simulink model "VehDyn14DOF"  (R2024b)
settings: Solver=VariableStepAuto  StartTime=0.0  StopTime=inf  FixedStep=0.001  RelTol=1e-3
model workspace (MAT data in the model file):
  ssEnable : Simulink.Parameter (value not decoded)
  xdot_r : Simulink.Parameter (value not decoded)
values from neighbouring files (symbols this model uses):
  AccPwrbp = 0.0 3.0779560993538198    [vehDyn14DOF.sldd]
  AccSpdbp = 256.49641719585139 641.24104298962845    [vehDyn14DOF.sldd]
  Downshift_Speeds = 9.5625 12.9375 16.3125 19.6875 23.0625 26.4375 29.8125 33.1875 36.5625 39.9375 43.3125 46.687499999999986 47.8125 51.187499999999986 54.562499999999986 57.9375 59.0625 62.4375 65.8125 69.1875 68.90625 72.84375 76.78125 80.71875 78.75 83.25 87.75 92.25    [vehDyn14DOF.sldd]
  EngRevLim = 7000.0    [vehDyn14DOF.sldd]
  F0z = 2886.0 2907.0    [vehDyn14DOF.sldd]
  Pedal_Positions = 0.1 0.4 0.5 0.9    [vehDyn14DOF.sldd]
  Trans = 0.01    [vehDyn14DOF.sldd]
  Upshift_Speeds = 12.9375 16.3125 19.6875 33.0 26.4375 29.8125 33.1875 52.5 39.9375 43.3125 46.687499999999986 77.25 51.187499999999986 54.562499999999986 57.9375 100.5 62.4375 65.8125 69.1875 138.75 72.84375 76.78125 80.71875 161.875 83.25 87.75 92.25 185.0    [vehDyn14DOF.sldd]
  VEH = 1575.0    [vehDyn14DOF.sldd]
symbols that are objects in the model workspace (value not decoded): ssEnable, xdot_r
undefined symbols (not defined in the file or in its folder): AccelCmd, CurvGradRef, CurvRef, DecelCmd, DiscIntNeverNeededParam, egoVehDyn, EnblAccelCmd, EnblDecelCmd, EnblSteerCmd, GearCmd, Gnd, Iz, lambda_mux, lambda_muy, lf, LngRef, lr, LtrRef, m, max_dc, maxSteer, PhiRef, SteerCmd, steeringGain, SteerZero, Wind, XRef, YRef, Z
libraries: simulink x14, autolibutils x13, autolibsharedcoupling x11, vehdynlibtire x10, vehdynlibsuspension x8, sharedtransform x5, autolibshareddiff x5, shared6dof x2, slpidlib x1, autolibtranscontrolscommon x1, vehdynlibdriver x1, autolibshared x1
(part 3 of 10)

== system VehDyn14DOF/Passenger Vehicle/Engine Input ==
  Cntrl : Inport
  Driveline : Inport  Port=2
  Bus Selector : BusSelector  OutputSignals=ECU.EngTrqCmd
  Bus Selector1 : BusSelector  OutputSignals=EngSpd
  EngTrqCmd : Outport  VectorParamsAs1DForOutWhenUnconnected=off
  EngSpd : Outport  Port=2  VectorParamsAs1DForOutWhenUnconnected=off
  wires:
  Driveline/1 -> Bus Selector1/1
  Cntrl/1 -> Bus Selector/1
  Bus Selector/1 -> EngTrqCmd/1  "<EngTrqCmd>"
  Bus Selector1/1 -> EngSpd/1  "<EngSpd>"

== system VehDyn14DOF/Passenger Vehicle/Engine Output ==
  "EngTrq " : Inport
  Bus Creator : BusCreator  Inputs=1
  Eng : Outport  VectorParamsAs1DForOutWhenUnconnected=off
  wires:
  "EngTrq "/1 -> Bus Creator/1  "EngTrq"
  Bus Creator/1 -> Eng/1

== system VehDyn14DOF/Passenger Vehicle/Pedal Cluster Input ==
  Driver : Inport
  Driveline : Inport  Port=2
  Steering : Inport  Port=3
  Bus Selector : BusSelector  OutputSignals=steer_cmd,accel_cmd,decel_cmd,gear_cmd
  Bus Selector1 : BusSelector  OutputSignals=BrkPrs
  Bus Selector2 : BusSelector  OutputSignals=StrWhlTrq
  SteerCmd : Outport  VectorParamsAs1DForOutWhenUnconnected=off
  AccelCmd : Outport  Port=2  VectorParamsAs1DForOutWhenUnconnected=off
  DecelCmd : Outport  Port=3  VectorParamsAs1DForOutWhenUnconnected=off
  GearCmd : Outport  Port=4  VectorParamsAs1DForOutWhenUnconnected=off
  BrkPrs : Outport  Port=5  VectorParamsAs1DForOutWhenUnconnected=off
  StrWhlTrq : Outport  Port=6  VectorParamsAs1DForOutWhenUnconnected=off
  wires:
  Bus Selector/2 -> AccelCmd/1  "<accel_cmd>"
  Driver/1 -> Bus Selector/1
  Bus Selector/3 -> DecelCmd/1  "<decel_cmd>"
  Bus Selector/4 -> GearCmd/1  "<gear_cmd>"
  Bus Selector/1 -> SteerCmd/1  "<steer_cmd>"
  Driveline/1 -> Bus Selector1/1
  Bus Selector1/1 -> BrkPrs/1  "<BrkPrs>"
  Steering/1 -> Bus Selector2/1
  Bus Selector2/1 -> StrWhlTrq/1  "<StrWhlTrq>"

== system VehDyn14DOF/Passenger Vehicle/Pedal Cluster Output ==
  SteerFdbk : Inport
  AccFdbk : Inport  Port=2
  DecelFdbk : Inport  Port=3
  GearFdbk : Inport  Port=4
  Bus Creator1 : BusCreator  Inputs=4
  Signal Specification : SignalSpecification  Unit=rad
  Signal Specification1 : SignalSpecification  Unit=1
  Signal Specification2 : SignalSpecification  Unit=1
  Signal Specification3 : SignalSpecification  Unit=1
  OperatorFdbk : Outport
  wires:
  Signal Specification1/1 -> Bus Creator1/2  "AccFdbk"
  Signal Specification3/1 -> Bus Creator1/4  "GearFdbk"
  AccFdbk/1 -> Signal Specification1/1
  DecelFdbk/1 -> Signal Specification2/1
  GearFdbk/1 -> Signal Specification3/1
  Signal Specification/1 -> Bus Creator1/1  "SteerFdbk"
  SteerFdbk/1 -> Signal Specification/1
  Bus Creator1/1 -> OperatorFdbk/1
  Signal Specification2/1 -> Bus Creator1/3  "DecelFdbk"

== system VehDyn14DOF/Passenger Vehicle/Pedal Cluster and Cabin ==
  note: Placeholder for introducing faults, detailed actuator behavior,
      | interactions of other systems with a human interface such
      | as changes in power steering and braking assistance.
  SteerCmd : Inport
  AccCmd : Inport  Port=2
  DecelCmd : Inport  Port=3
  GearCmd : Inport  Port=4
  BrkPrs : Inport  Port=5
  StrWhlTrq : Inport  Port=6
  Brake Pedal : Subsystem
  Dead Zone2 : DeadZone  LowerValue=0  UpperValue=.01  ZeroCross=off
  Dead Zone3 : DeadZone  LowerValue=-.01  UpperValue=.01  ZeroCross=off
  Terminator : Terminator
  Terminator1 : Terminator
  SteerFdbk : Outport
  AccFdbk : Outport  Port=2
  DecelFdbk : Outport  Port=3
  GearFdbk : Outport  Port=4
  wires:
  SteerCmd/1 -> Dead Zone3/1
  AccCmd/1 -> Dead Zone2/1
  DecelCmd/1 -> Brake Pedal/1(DecelCmd)
  GearCmd/1 -> GearFdbk/1
  BrkPrs/1 -> Terminator/1
  StrWhlTrq/1 -> Terminator1/1
  Brake Pedal/1(DecelFdbk) -> DecelFdbk/1
  Dead Zone2/1 -> AccFdbk/1
  Dead Zone3/1 -> SteerFdbk/1

== system VehDyn14DOF/Passenger Vehicle/Steering and Driveline ==
  SteerHWCmd : Inport
  EngTrq : Inport  Port=2
  GearCmd : Inport  Port=3  OutDataTypeStr=int8
  BrkPrsCmd : Inport  Port=4  PortDimensions=4
  Omega : Inport  Port=5
  DiffPrsCmd : Inport  Port=6
  Brake Hydraulics : Subsystem
  Bus Selector : BusSelector  OutputSignals=Trans.TransGear
  Constant : Constant  Value=0
  Driveline Model : Subsystem  Variant=on  VariantControlMode=label  LabelModeActiveChoice=4
  Ground : Ground
  Kinematic Steering : vehdynlibsteering/Kinematic Steering  StrgType=Ackerman  StrgRatioType=Constant  Loc=Front  NrmlFctr=1  TrckWdth=1.922  WhlBase=lf+lr  Db=0  StrgRng=maxSteer*18  StrgAngBpts="[-6.2832   -5.0265   -3.7699   -2.5133   -1.2566         0    1.2566    2.5133    3.7699    5.0265    6.2832]"  StrgRatioTbl=|  StrgRatio=18  PctAckIn=off  PctAck=100  PctAckTbl=ones(1,11)*100  StrgArmLngth=0.1  RckCsLngth=0.5  TieRodLngth=0.248128028933392  D=0.2  PnnRadius=0.0057  PnnRadiusTbl="[0.0055    0.0055    0.0056    0.0057    0.0057    0.0057    0.0057    0.0057    0.0056    0.0055    0.0055]"  RodLngth=0.1  ParaArmLngth=0.9  aMode=2
      | [13.5000   13.3750   13.2500   13.1250   13.0000   13.0000   13.0000   13.1250   13.2500   13.3750   13.5000
      | ]
  Terminator : Terminator
  Transmission : Subsystem  Variant=on  VariantControlMode=label  LabelModeActiveChoice=0
  Vector Concatenate : Concatenate
  Vector Concatenate1 : Concatenate
  Vector Concatenate2 : Concatenate
  WhlAng : Outport  Unit=rad  VectorParamsAs1DForOutWhenUnconnected=off
  AxlTrq : Outport  Port=2  VectorParamsAs1DForOutWhenUnconnected=off
  BrkPrs : Outport  Port=3  PortDimensions=4  VectorParamsAs1DForOutWhenUnconnected=off
  EngSpd : Outport  Port=4  Unit=rad/s  VectorParamsAs1DForOutWhenUnconnected=off
  PropShftSpd : Outport  Port=5  VectorParamsAs1DForOutWhenUnconnected=off
  StrWhlTrq : Outport  Port=6  Unit=N*m  VectorParamsAs1DForOutWhenUnconnected=off
  Gear : Outport  Port=7  Unit=1  VectorParamsAs1DForOutWhenUnconnected=off
  wires:
  Driveline Model/1(AxlTrq) -> AxlTrq/1
  SteerHWCmd/1 -> Kinematic Steering/1
  Driveline Model/2(PropShaftSpd) -> PropShftSpd/1, Transmission/3(PropShftSpd)
  BrkPrsCmd/1 -> Brake Hydraulics/1(BrkPrsCmd)
  Kinematic Steering/2 -> Vector Concatenate/1
  Transmission/3(DrvShfTrq) -> Driveline Model/1(DrvShfTrq)
  Transmission/1(Info) -> Bus Selector/1
  Bus Selector/1 -> Gear/1  "<TransGear>"
  Kinematic Steering/3 -> Vector Concatenate/2
  Vector Concatenate2/1 -> Vector Concatenate1/2  "RearWheelAngles"
  Ground/1 -> StrWhlTrq/1
  DiffPrsCmd/1 -> Driveline Model/3(DiffPrsCmd)
  Brake Hydraulics/1(BrkPrs) -> BrkPrs/1
  Kinematic Steering/1 -> Terminator/1
  EngTrq/1 -> Transmission/2(EngTrq)
  Omega/1 -> Driveline Model/2(Omega)
  Vector Concatenate/1 -> Vector Concatenate1/1  "FrontWheelAngles"
  Transmission/2(EngSpd) -> EngSpd/1
  GearCmd/1 -> Transmission/1(GearCmd)
  Vector Concatenate1/1 -> WhlAng/1
  Constant/1 -> Vector Concatenate2/1, Vector Concatenate2/2

== system VehDyn14DOF/Controllers/Active Differential Control/No Control ==
  axayaz : Inport
  Steer : Inport  Port=2
  Constant : Constant  Value=0
  Constant1 : Constant  Value=0
  Terminator : Terminator
  Terminator1 : Terminator
  Vector Concatenate2 : Concatenate  NumInputs=4
  DiffPrsCmd : Outport  VectorParamsAs1DForOutWhenUnconnected=off
  TrqCmd : Outport  Port=2  VectorParamsAs1DForOutWhenUnconnected=off
  wires:
  Constant/1 -> Vector Concatenate2/1, Vector Concatenate2/4, Vector Concatenate2/3, Vector Concatenate2/2
  Steer/1 -> Terminator1/1
  Vector Concatenate2/1 -> DiffPrsCmd/1  "DiffPrsCmd"
  axayaz/1 -> Terminator/1
  Constant1/1 -> TrqCmd/1  "TrqCmd"

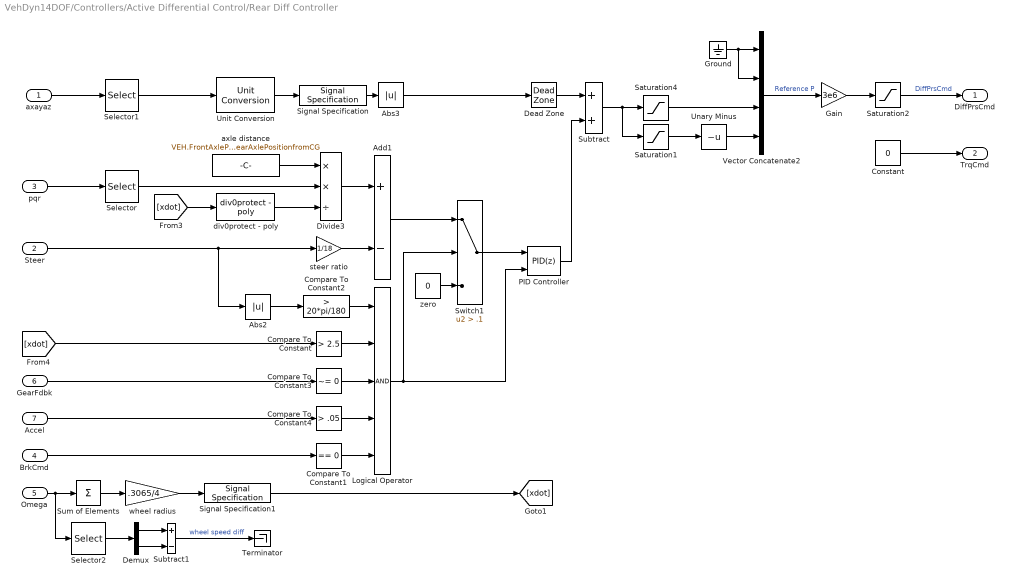
== system VehDyn14DOF/Controllers/Active Differential Control/Rear Diff Controller ==
  axayaz : Inport
  Steer : Inport  Port=2
  pqr : Inport  Port=3
  BrkCmd : Inport  Port=4
  Omega : Inport  Port=5  Unit=rad/s
  GearFdbk : Inport  Port=6
  Accel : Inport  Port=7
  Abs2 : Abs  SaturateOnIntegerOverflow=off
  Abs3 : Abs  ZeroCross=off  SaturateOnIntegerOverflow=off
  Add1 : Sum  Inputs=+-
  Compare To Constant : simulink/Logic and Bit Operations/Compare To Constant  relop=>  const=2.5  OutDataTypeStr=boolean
  Compare To Constant1 : simulink/Logic and Bit Operations/Compare To Constant  relop===  const=0  OutDataTypeStr=boolean
  Compare To Constant2 : simulink/Logic and Bit Operations/Compare To Constant  relop=>  const=20*pi/180  OutDataTypeStr=boolean
  Compare To Constant3 : simulink/Logic and Bit Operations/Compare To Constant  relop=~=  const=0  OutDataTypeStr=boolean
  Compare To Constant4 : simulink/Logic and Bit Operations/Compare To Constant  relop=>  const=.05  OutDataTypeStr=boolean
  Constant : Constant  Value=0
  Dead Zone : DeadZone  ZeroCross=off
  Demux : Demux  Outputs=2
  Divide3 : Product  Inputs=**/
  Gain : Gain  Gain=3e6
  Ground : Ground
  Logical Operator : Logic  Inputs=5  AllPortsSameDT=off  OutDataTypeStr=boolean
  PID Controller : slpidlib/PID Controller  Controller=PID  Form=Parallel  TimeDomain=Discrete-time  UseExternalTs=off  SampleTime=-1  IntegratorMethod=Forward Euler  FilterMethod=Forward Euler  ControllerParametersSource=internal  P=1  I=.05  UseKiTs=off  D=0  UseExternalDerivativeSource=off  N=1  UseFilter=on  TunerSelectOption=Transfer Function Based (PID Tuner App)  ZeroCross=off  InitialConditionSource=internal  InitialConditionForIntegrator=0  InitialConditionForFilter=0  DifferentiatorICPrevScaledInput=0  ExternalReset=either  TrackingMode=off  Kt=1  LimitOutput=on  SatLimitsSource=internal  UpperSaturationLimit=1  LowerSaturationLimit=-1  LinearizeAsGain=on  AntiWindupMode=clamping  Kb=1  LimitIntegrator=off  UpperIntegratorSaturationLimit=inf  LowerIntegratorSaturationLimit=-inf  POutMin=[]  POutMax=[]  IOutMin=[]  IOutMax=[]  DOutMin=[]  DOutMax=[]  NOutMin=[]  NOutMax=[]  SumOutMin=[]  SumOutMax=[]  SaturationOutMin=[]  SaturationOutMax=[]  PParamMin=[]  PParamMax=[]  IParamMin=[]  IParamMax=[]  DParamMin=[]  DParamMax=[]  NParamMin=[]  NParamMax=[]  KbParamMin=[]  KbParamMax=[]  KtParamMin=[]  KtParamMax=[]  KbOutMin=[]  KbOutMax=[]  KtOutMin=[]  KtOutMax=[]  IntegratorOutMin=[]  IntegratorOutMax=[]  FilterOutMin=[]  FilterOutMax=[]  SumI1OutMin=[]  SumI1OutMax=[]  SumI2OutMin=[]  SumI2OutMax=[]  SumI3OutMin=[]  SumI3OutMax=[]  SumI4OutMin=[]  SumI4OutMax=[]  SumDOutMin=[]  SumDOutMax=[]  DifferentiatorOutMin=[]  DifferentiatorOutMax=[]  FilterDiffOutCoefMin=[]  FilterDiffOutCoefMax=[]  ReciprocalOutMin=[]  ReciprocalOutMax=[]  SumDenOutMin=[]  SumDenOutMax=[]  SumNumOutMin=[]  SumNumOutMax=[]  DivideOutMin=[]  DivideOutMax=[]  UdiffTsProdOutMin=[]  UdiffTsProdOutMax=[]  NTsProdOutMin=[]  NTsProdOutMax=[]  UintegralTsProdOutMin=[]  UintegralTsProdOutMax=[]  UngainTsProdOutMin=[]  UngainTsProdOutMax=[]  ClampingZeroOutDataTypeStr=Inherit: Inherit via back propagation  ClampingZeroOutMin=[]  ClampingZeroOutMax=[]  FilterDenConstantOutDataTypeStr=Inherit: Inherit via back propagation  FilterDenConstantOutMin=[]  FilterDenConstantOutMax=[]  PCopyOutDataTypeStr=Inherit: Inherit via back propagation  PCopyOutMin=[]  PCopyOutMax=[]  NCopyOutDataTypeStr=Inherit: Inherit via back propagation  NCopyOutMin=[]  NCopyOutMax=[]  IntegratorContinuousStateAttributes=''  IntegratorStateMustResolveToSignalObject=off  IntegratorRTWStateStorageClass=Auto  FilterContinuousStateAttributes=''  FilterStateMustResolveToSignalObject=off  FilterRTWStateStorageClass=Auto  ParallelPVariant=InternalParameters  IdealPVariant=Disabled  IVariant=InternalParameters  DVariant=InternalParameters  IntegratorVariant=Discrete  SatVariant=Enabled  AWVariant=DiscClampingParallel  PCopyVariant=Disabled  TRVariant=Disabled  FdbkBlocksVariant=Forward  IdealPFdbkVariant=Disabled  SatFdbkVariant=Disabled  DerivativeFilterVariant=ForwardEulerFilter  NVariant=InternalParameters  NCopyVariant=Disabled  FilterICVariant=InternalICsFilter  IntegratorICVariant=InternalICs  ExternalResetVariant=ExternalReset  TRSumVariant=Passthrough  SumFdbkVariant=Disabled  SumVariant=Sum_PID  TsampFilterVariant=InternalTs  TsampNgainVariant=Passthrough  TsampIntegralVariant=Disabled_SignalSpec  ExternalSaturationOutDataTypeStr=Inherit: Same as second input  DerivativeSourceVariant=ErrorSignal  PreIntVariant=InternalPreInt
  Saturation1 : Saturate  UpperLimit=0  LowerLimit=-1  ZeroCross=off
  Saturation2 : Saturate  UpperLimit=5e6  LowerLimit=0  ZeroCross=off
  Saturation4 : Saturate  UpperLimit=1  LowerLimit=0  ZeroCross=off
  Selector : Selector  InputPortWidth=3  IndexOptions=Index vector (dialog)  Indices=[3]  OutputSizes=1
  Selector1 : Selector  InputPortWidth=3  IndexOptions=Index vector (dialog)  Indices=[2]  OutputSizes=1
  Selector2 : Selector  InputPortWidth=4  IndexOptions=Index vector (dialog)  Indices=[3 4]  OutputSizes=1
  Signal Specification : SignalSpecification  Unit=gn
  Signal Specification1 : SignalSpecification  Unit=m/s
  Subtract : Sum
  Subtract1 : Sum  Inputs=+-
  Sum of Elements : Sum  Inputs=+
  Switch1 : Switch  Criteria=u2 > Threshold  Threshold=.1  SaturateOnIntegerOverflow=off  InputSameDT=off
  Terminator : Terminator
  Unary Minus : UnaryMinus
  Unit Conversion : UnitConversion
  Vector Concatenate2 : Concatenate  NumInputs=4
  axle distance : Constant  Value=VEH.FrontAxlePositionfromCG+VEH.RearAxlePositionfromCG
  div0protect - poly : autolibutils/div0protect - poly  thresh=1  ZeroCross1=on  aMode=2
  steer ratio : Gain  Gain=1/18
  wheel radius : Gain  Gain=.3065/4
  zero : Constant  Value=0
  DiffPrsCmd : Outport  VectorParamsAs1DForOutWhenUnconnected=off
  TrqCmd : Outport  Port=2  VectorParamsAs1DForOutWhenUnconnected=off
  wires:
  Vector Concatenate2/1 -> Gain/1  "Reference P"
  Ground/1 -> Vector Concatenate2/2, Vector Concatenate2/1
  Saturation1/1 -> Unary Minus/1
  Gain/1 -> Saturation2/1
  Saturation2/1 -> DiffPrsCmd/1  "DiffPrsCmd"
  Divide3/1 -> Add1/1
  Selector/1 -> Divide3/2
  Logical Operator/1 -> PID Controller/2, Switch1/2
  Switch1/1 -> PID Controller/1
  zero/1 -> Switch1/3
  PID Controller/1 -> Subtract/2
  Add1/1 -> Switch1/1
  axle distance/1 -> Divide3/1
  pqr/1 -> Selector/1
  Compare To Constant2/1 -> Logical Operator/1
  Compare To Constant/1 -> Logical Operator/2
  Abs2/1 -> Compare To Constant2/1
  Steer/1 -> Abs2/1, steer ratio/1
  [xdot] -> Compare To Constant/1
  axayaz/1 -> Selector1/1
  Sum of Elements/1 -> wheel radius/1
  wheel radius/1 -> Signal Specification1/1
  Omega/1 -> Selector2/1, Sum of Elements/1
  Signal Specification1/1 -> [xdot]
  BrkCmd/1 -> Compare To Constant1/1
  GearFdbk/1 -> Compare To Constant3/1
  Compare To Constant3/1 -> Logical Operator/3
  Subtract/1 -> Saturation1/1, Saturation4/1
  Accel/1 -> Compare To Constant4/1
  Compare To Constant4/1 -> Logical Operator/4
  steer ratio/1 -> Add1/2
  Saturation4/1 -> Vector Concatenate2/3
  Selector1/1 -> Unit Conversion/1
  Signal Specification/1 -> Abs3/1
  Abs3/1 -> Dead Zone/1
  Dead Zone/1 -> Subtract/1
  Constant/1 -> TrqCmd/1
  Selector2/1 -> Demux/1
  Demux/1 -> Subtract1/1
  Demux/2 -> Subtract1/2
  Unary Minus/1 -> Vector Concatenate2/4
  Subtract1/1 -> Terminator/1  "wheel speed diff"
  Compare To Constant1/1 -> Logical Operator/5
  Unit Conversion/1 -> Signal Specification/1
  [xdot] -> div0protect - poly/1
  div0protect - poly/1 -> Divide3/3

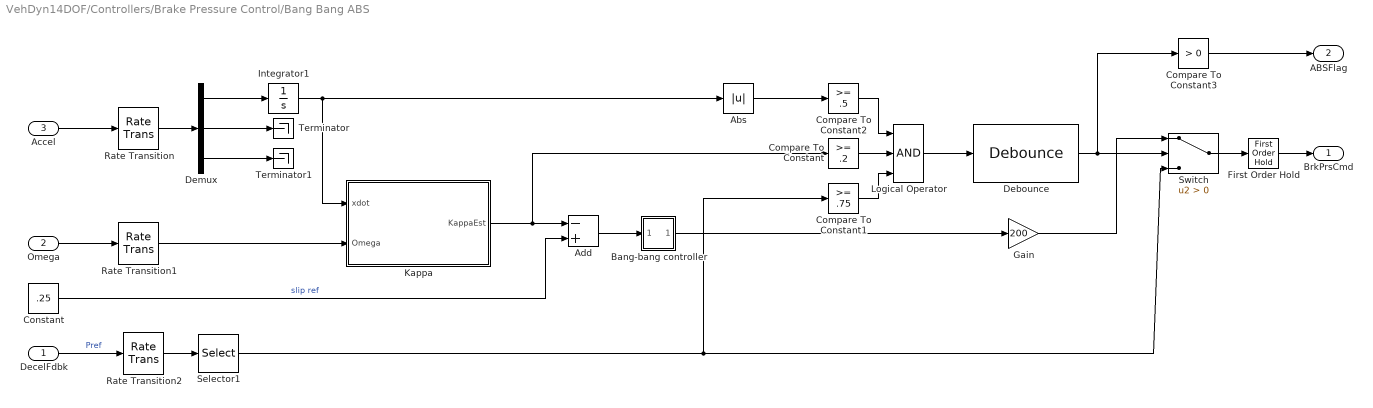
== system VehDyn14DOF/Controllers/Brake Pressure Control/Bang Bang ABS ==
  DecelFdbk : Inport
  Omega : Inport  Port=2
  Accel : Inport  Port=3
  Abs : Abs  SaturateOnIntegerOverflow=off
  Add : Sum  Inputs=-+
  Bang-bang controller : Subsystem  mask(Sign){}
      mask help: y = sign(x)
      mask Help: Sign Function:\n\t\t\ty = 1 if x > 0\n\t\t\ty = 0 if x = 0\n\t\t\ty = -1 if x < 0
      mask Display: plot(-50,-50,50,50,[-50,50],[0,0],[0,0],[-50,50],[-40,0],[-30,-30],[0,40],[30,30])
  Compare To Constant : simulink/Logic and Bit Operations/Compare To Constant  relop=>=  const=.2  OutDataTypeStr=boolean
  Compare To Constant1 : simulink/Logic and Bit Operations/Compare To Constant  relop=>=  const=.75  OutDataTypeStr=boolean
  Compare To Constant2 : simulink/Logic and Bit Operations/Compare To Constant  relop=>=  const=.5  OutDataTypeStr=boolean
  Compare To Constant3 : simulink/Logic and Bit Operations/Compare To Constant  relop=>  const=0  OutDataTypeStr=boolean  ZeroCross=off
  Constant : Constant  Value=.25
  Debounce : autolibutils/Debounce  DbcOn_Cnts=.1*.001  DbcOff_Cnts=.1*.001  aMode=2
  Demux : Demux  Outputs=3
  First Order Hold : FirstOrderHold  ErrorTolerance=1
  Gain : Gain  Gain=200
  Integrator1 : Integrator
  Kappa : Subsystem  TreatAsAtomicUnit=on
  Logical Operator : Logic  Inputs=3  AllPortsSameDT=off  OutDataTypeStr=boolean
  Rate Transition : RateTransition  Deterministic=off  OutPortSampleTime=.001
  Rate Transition1 : RateTransition  Deterministic=off  OutPortSampleTime=.001
  Rate Transition2 : RateTransition  Deterministic=off  OutPortSampleTime=.001
  Selector1 : Selector  InputPortWidth=1  IndexOptions=Index vector (dialog)  Indices=[1 1 1 1]  OutputSizes=1
  Switch : Switch  Criteria=u2 > Threshold  ZeroCross=off  SaturateOnIntegerOverflow=off  InputSameDT=off
  Terminator : Terminator
  Terminator1 : Terminator
  BrkPrsCmd : Outport  VectorParamsAs1DForOutWhenUnconnected=off
  ABSFlag : Outport  Port=2
  wires:
  Bang-bang controller/1(out_1) -> Gain/1
  Add/1 -> Bang-bang controller/1(in_1)
  First Order Hold/1 -> BrkPrsCmd/1
  DecelFdbk/1 -> Rate Transition2/1  "Pref"
  Constant/1 -> Add/2  "slip ref"
  Switch/1 -> First Order Hold/1
  Kappa/1(KappaEst) -> Add/1, Compare To Constant/1
  Logical Operator/1 -> Debounce/1
  Compare To Constant/1 -> Logical Operator/2
  Compare To Constant1/1 -> Logical Operator/3
  Debounce/1 -> Compare To Constant3/1, Switch/2
  Abs/1 -> Compare To Constant2/1
  Compare To Constant2/1 -> Logical Operator/1
  Gain/1 -> Switch/1
  Integrator1/1 -> Kappa/1(xdot), Abs/1
  Demux/2 -> Terminator/1
  Accel/1 -> Rate Transition/1
  Demux/1 -> Integrator1/1
  Rate Transition/1 -> Demux/1
  Demux/3 -> Terminator1/1
  Omega/1 -> Rate Transition1/1
  Rate Transition1/1 -> Kappa/2(Omega)
  Rate Transition2/1 -> Selector1/1
  Compare To Constant3/1 -> ABSFlag/1
  Selector1/1 -> Compare To Constant1/1, Switch/3

== system VehDyn14DOF/Controllers/Brake Pressure Control/Five-State ABS ==
  DecelFdbk : Inport
  Omega : Inport  Port=2
  Accel : Inport  Port=3
  ABSCtrlForEach : Subsystem  mask(Five-State ABS Control){Re=0.323, KappaOpt=-0.12, WhlAccelOpt=[-11, -11, -20, -20], v1=-0.3, v5=0.05, v4=0.3, a2=4, b=4, A=6.5, a1=4.5, aMode=2}
      mask prompts: Re "Wheel effective radius, Re [m]:"; KappaOpt "Desired wheel slip ratio, KappaOpt [-]:"; WhlAccelOpt "Desired wheel acceleration, WhlAccelOpt [m/s^2]:"; v1 "Braking pressure declining rate, v1 [-]:"; v5 "Secondary braking pressure rising rate, v5 [-]:"; v4 "Braking pressure rising rate, v4 [-]:"; a2 "Threshold of State 1, a2 [m/s^2]:"; b "Threshold of State 2, b [m/s^2]:"; A "Threshold of State 3 and 4, A [m/s^2]:"; a1 "Threshold of State 5, a1 [m/s^2]:"
      mask help: This block determines brake pressure varying rate for each wheel once the ABS controller is activated. During ABS control, only wheel speed is directly regulated.
      mask init:
      | [~]=vehdynicon('vehdynblk',gcb);
      mask DialogControl vehParamGroup Prompt: Vehicle Parameter
      mask DialogControl ParameterGroupVar Prompt: Desired Control Parameters
      mask DialogControl Container3 Prompt: Braking Pressure Rates
      mask DialogControl Container4 Prompt: Wheel Acceleration Thresholds
  First Order Hold : FirstOrderHold  ErrorTolerance=0.1
  First Order Hold1 : FirstOrderHold  ErrorTolerance=1
  Rate Transition : RateTransition  OutPortSampleTime=.001
  Rate Transition1 : RateTransition  OutPortSampleTime=.001
  Rate Transition2 : RateTransition  OutPortSampleTime=.001
  Wheel Accel and Slip Estimator : Subsystem
  BrkPrsCmd : Outport
  ABSFlag : Outport  Port=2  PortDimensions=4
  wires:
  Omega/1 -> Rate Transition1/1
  Accel/1 -> Rate Transition2/1
  DecelFdbk/1 -> Rate Transition/1
  Wheel Accel and Slip Estimator/1(<WhlAccel>) -> ABSCtrlForEach/2(WhlAccel)
  Wheel Accel and Slip Estimator/2(<Kappa>) -> ABSCtrlForEach/3(WhlSlip)
  Wheel Accel and Slip Estimator/3(<xdot>) -> ABSCtrlForEach/4(VehSpd)
  ABSCtrlForEach/2(BrkFlag) -> First Order Hold1/1
  First Order Hold/1 -> BrkPrsCmd/1
  Rate Transition/1 -> ABSCtrlForEach/1(Pref)
  Rate Transition1/1 -> Wheel Accel and Slip Estimator/1(Omega)
  Rate Transition2/1 -> Wheel Accel and Slip Estimator/2(Accel)
  First Order Hold1/1 -> ABSFlag/1
  ABSCtrlForEach/1(BrkCtrl) -> First Order Hold/1

== system VehDyn14DOF/Controllers/Brake Pressure Control/Open Loop ==
  DecelFdbk : Inport
  Constant : Constant  Value=false
  Selector : Selector  InputPortWidth=1  IndexOptions=Index vector (dialog)  Indices=[1 1 1 1]  OutputSizes=1
  Selector1 : Selector  InputPortWidth=1  IndexOptions=Index vector (dialog)  Indices=[1 1 1 1]  OutputSizes=1
  BrkPrsCmd : Outport  VectorParamsAs1DForOutWhenUnconnected=off
  ABSFlag : Outport  Port=2
  wires:
  DecelFdbk/1 -> Selector1/1
  Selector1/1 -> BrkPrsCmd/1
  Constant/1 -> Selector/1
  Selector/1 -> ABSFlag/1

== system VehDyn14DOF/Controllers/ECU/Torque Cmd ==
  DiffTrqCmd : Inport
  <Accel> : Inport  Port=2
  EngSpd : Inport  Port=3
  ABSFlag : Inport  Port=4
  Acc to Torque Request : Gain  Gain=150
  Constant : Constant  Value=0
  Max : MinMax  Function=max  Inputs=2
  OR : Logic  Operator=OR  Inputs=1  AllPortsSameDT=off  OutDataTypeStr=boolean
  Rev Limiter Control : Subsystem
  Signal Specification : SignalSpecification  Unit=rpm
  Switch : Switch  Criteria=u2 > Threshold  ZeroCross=off  SaturateOnIntegerOverflow=off  InputSameDT=off
  Unit Conversion : UnitConversion
  EngTrqCmd : Outport
  wires:
  Signal Specification/1 -> Rev Limiter Control/2(EngSpd)  "EngSpd"
  Unit Conversion/1 -> Signal Specification/1
  EngSpd/1 -> Unit Conversion/1
  <Accel>/1 -> Acc to Torque Request/1
  Acc to Torque Request/1 -> Rev Limiter Control/1(TrqCmd)
  DiffTrqCmd/1 -> Max/1
  Rev Limiter Control/1(TrqCmdRevLimited) -> Max/2
  Switch/1 -> EngTrqCmd/1
  Max/1 -> Switch/3
  ABSFlag/1 -> OR/1
  Constant/1 -> Switch/1
  OR/1 -> Switch/2

== system VehDyn14DOF/Controllers/Transmission Controller/Driver - No Clutch ==
  GearReq : Inport
  Gear : Outport  VectorParamsAs1DForOutWhenUnconnected=off
  wires:
  GearReq/1 -> Gear/1

== system VehDyn14DOF/Controllers/Transmission Controller/PRNDL Controller ==
  Accel : Inport
  BrkCmd : Inport  Port=2
  Omega : Inport  Port=3  Unit=rad/s
  EngSpd : Inport  Port=4  Unit=rad/s
  GearReq : Inport  Port=5
  ABSFlag : Inport  Port=6
  Gain : Gain  Gain=0.3/4
  OR : Logic  Operator=OR  Inputs=1  AllPortsSameDT=off  OutDataTypeStr=boolean
  Signal Specification : SignalSpecification  Unit=m/s
  Sum of Elements : Sum  Inputs=+
  Transmission Controller PRNDL : autolibtranscontrolscommon/Transmission Controller PRNDL  DriveMode=off  GearInit=0  LugSpd=1200  MinUpSpd=1000  tClutchUp=0.5  tClutchDn=0.5  tPark=120  VelUnit=km/hr  UpShSpd=|  UpLdBpt=[0.1 0.4 0.5 0.9]  UpShBpt=1:7  UpPtBpt=[1 2]  DnShfSpd=|  DnShSpd=[9.5625 23.0625 36.5625 47.8125 59.0625 68.90625 78.75;12.9375 26.4375 39.9375 51.187499999999986 62.4375 72.84375 83.25;16.3125 29.8125 43.3125 54.562499999999986 65.8125 76.78125 87.75;19.6875 33.1875 46.687499999999986 57.9375 69.1875 80.71875 92.25]  DnLdBpt=[0.1 0.4 0.5 0.9]  DnShBpt=2:8  DnPtBpt=[1 2]  POFS=zeros(4,1)  GOFS=zeros(1,7)  Ngears=8  aMode=6
      UpShSpd=|
      | reshape([35.6199
      |    40.1199
      |    41.6199
      |    47.6199
      |    48.3186
      |    52.8186
      |    54.3186
      |    60.3186
      |    57.5984
      |    62.0984
      |    63.5984
      |    69.5984
      |    70.2526
      |    74.7526
      |    76.2526
      |    82.2526
      |    88.5310
      |    93.0310
      |    94.5310
      |   100.5310
      |   138.7964
      |   143.2964
      |   144.7964
      |   150.7964
      |   214.1947
      |   218.6947
      |   220.1947
      |   226.1947
      |    35.6199
      |    40.1199
      |    41.6199
      |    47.6199
      |    48.3186
      |    52.8186
      |    54.3186
      |    60.3186
      |    57.5984
      |    62.0984
      |    63.5984
      |    69.5984
      |    70.2526
      |    74.7526
      |    76.2526
      |    82.2526
      |    88.5310
      |    93.0310
      |    94.5310
      |   100.5310
      |   138.7964
      |   143.2964
      |   144.7964
      |   150.7964
      |   214.1947
      |   218.6947
      |   220.1947
      |   226.1947],4,7,2)
      DnShfSpd=|
      | reshape([31.6199
      |    36.1199
      |    37.6199
      |    43.6199
      |    44.3186
      |    48.8186
      |    50.3186
      |    56.3186
      |    53.5984
      |    58.0984
      |    59.5984
      |    65.5984
      |    66.2526
      |    70.7526
      |    72.2526
      |    78.2526
      |    84.5310
      |    89.0310
      |    90.5310
      |    96.5310
      |   134.7964
      |   139.2964
      |   140.7964
      |   146.7964
      |   210.1947
      |   214.6947
      |   216.1947
      |   222.1947
      |    31.6199
      |    36.1199
      |    37.6199
      |    43.6199
      |    44.3186
      |    48.8186
      |    50.3186
      |    56.3186
      |    53.5984
      |    58.0984
      |    59.5984
      |    65.5984
      |    66.2526
      |    70.7526
      |    72.2526
      |    78.2526
      |    84.5310
      |    89.0310
      |    90.5310
      |    96.5310
      |   134.7964
      |   139.2964
      |   140.7964
      |   146.7964
      |   210.1947
      |   214.6947
      |   216.1947
      |   222.1947],4,7,2)
  Gear : Outport  VectorParamsAs1DForOutWhenUnconnected=off
  wires:
  Transmission Controller PRNDL/1 -> Gear/1
  EngSpd/1 -> Transmission Controller PRNDL/5
  GearReq/1 -> Transmission Controller PRNDL/1
  Omega/1 -> Sum of Elements/1
  ABSFlag/1 -> OR/1
  BrkCmd/1 -> Transmission Controller PRNDL/3
  Accel/1 -> Transmission Controller PRNDL/2
  OR/1 -> Transmission Controller PRNDL/6
  Gain/1 -> Signal Specification/1
  Signal Specification/1 -> Transmission Controller PRNDL/4
  Sum of Elements/1 -> Gain/1

== system VehDyn14DOF/Controllers/Transmission Controller/Paddles ==
  Accel : Inport
  EngSpd : Inport  Port=2  Unit=rad/s
  Add1 : Sum  Inputs=+-+
  Current Gear : UnitDelay  SampleTime=-1  HasFrameUpgradeWarning=on
  Data Type Conversion2 : DataTypeConversion  OutDataTypeStr=double  SaturateOnIntegerOverflow=off  RndMeth=Floor
  Debounce : autolibutils/Debounce  DbcOn_Cnts=10  DbcOff_Cnts=10  aMode=aMode
  Debounce1 : autolibutils/Debounce  DbcOn_Cnts=10  DbcOff_Cnts=10  aMode=aMode
  Demux : Demux  Outputs=2
  Detect Increase2 : simulink/Logic and Bit Operations/Detect Increase  vinit=0.0  OutDataTypeStr=boolean
  Logical Operator1 : Logic  Operator=XOR  Inputs=1  AllPortsSameDT=off  OutDataTypeStr=boolean
  Mux : Mux  Inputs=2
  Switch2 : Switch  Criteria=u2 > Threshold  SaturateOnIntegerOverflow=off  InputSameDT=off
  Gear : Outport  VectorParamsAs1DForOutWhenUnconnected=off
  wires:
  Debounce/1 -> Mux/1
  Mux/1 -> Detect Increase2/1
  Logical Operator1/1 -> Switch2/2
  Data Type Conversion2/1 -> Demux/1
  Demux/1 -> Add1/1
  Demux/2 -> Add1/2
  Current Gear/1 -> Add1/3, Switch2/3
  Switch2/1 -> Gear/1, Current Gear/1
  Debounce1/1 -> Mux/2
  Add1/1 -> Switch2/1
  Detect Increase2/1 -> Data Type Conversion2/1, Logical Operator1/1
  EngSpd/1 -> Debounce1/1
  Accel/1 -> Debounce/1

== system VehDyn14DOF/Controllers/Transmission Controller/Transmission Controller ==
  Accel : Inport
  EngSpd : Inport  Port=2  Unit=rad/s
  Omega : Inport  Port=3  Unit=rad/s
  10ms Function-Call Generator : simulink/Ports & Subsystems/Function-Call Generator  sample_time=0.01  numberOfIterations=1  DisallowWideOutput=off
  Data Type Conversion : DataTypeConversion  SaturateOnIntegerOverflow=off  RndMeth=Floor
  First Order Hold : FirstOrderHold  ErrorTolerance=.1
  Rate Transition : RateTransition  Deterministic=off
  Rate Transition1 : RateTransition  Deterministic=off
  Rate Transition2 : RateTransition  Deterministic=off
  Signal Specification : SignalSpecification  Unit=rpm
  TCM : Subsystem
  Unit Conversion : UnitConversion
  Gear : Outport  VectorParamsAs1DForOutWhenUnconnected=off
  wires:
  TCM/1(GearCmd) -> Data Type Conversion/1
  Rate Transition/1 -> TCM/1(AccCmd)
  10ms Function-Call Generator/1 -> TCM/Trigger
  Accel/1 -> Rate Transition/1
  Omega/1 -> Rate Transition2/1
  Rate Transition1/1 -> TCM/2(EngSpd)
  First Order Hold/1 -> Gear/1
  Unit Conversion/1 -> Signal Specification/1
  Signal Specification/1 -> Rate Transition1/1  "EngSpd"
  EngSpd/1 -> Unit Conversion/1
  Data Type Conversion/1 -> First Order Hold/1
  Rate Transition2/1 -> TCM/3(Omega)

== system VehDyn14DOF/Passenger Vehicle/Chassis and Tires/Suspension ==
  Steering : Inport
  Vehicle : Inport  Port=2
  Wheel : Inport  Port=3
  Double Wishbone Suspension : Subsystem  VariantControl=1
      mask Display: image('suspdw.png');
  Independent Mapped Front Suspension Mapped Solid Axle Rear Suspension : Subsystem  VariantControl=2
      mask Display: image([imread('suspindmap.png');imread('suspsamap.png')]);
  Kinematics and Compliance Independent Suspension : Subsystem  VariantControl=6
      mask Display: image('suspkandc.png');
  MacPherson Front Suspension Solid Axle Rear Suspension : Subsystem  VariantControl=3
      mask Display: image([imread('suspmacp.png');imread('suspsacoil.png')]);
  MacPherson Suspension : Subsystem  VariantControl=4
      mask Display: image('suspmacp.png');
  Mapped Suspension : Subsystem  VariantControl=5
      mask Display: image('suspindmap.png');
  Suspension : Outport  VectorParamsAs1DForOutWhenUnconnected=off

== system VehDyn14DOF/Passenger Vehicle/Chassis and Tires/Vehicle ==
  Suspension : Inport
  Wind : Inport  Port=2
  Variant Subsystem : Subsystem  Variant=on  VariantControlMode=label  LabelModeActiveChoice=1
  VehFdbk : Outport  VectorParamsAs1DForOutWhenUnconnected=off
  wires:
  Variant Subsystem/1(VehFdbk) -> VehFdbk/1  "VehFdbk"
  Wind/1 -> Variant Subsystem/2(Wind)
  Suspension/1 -> Variant Subsystem/1(Suspension)

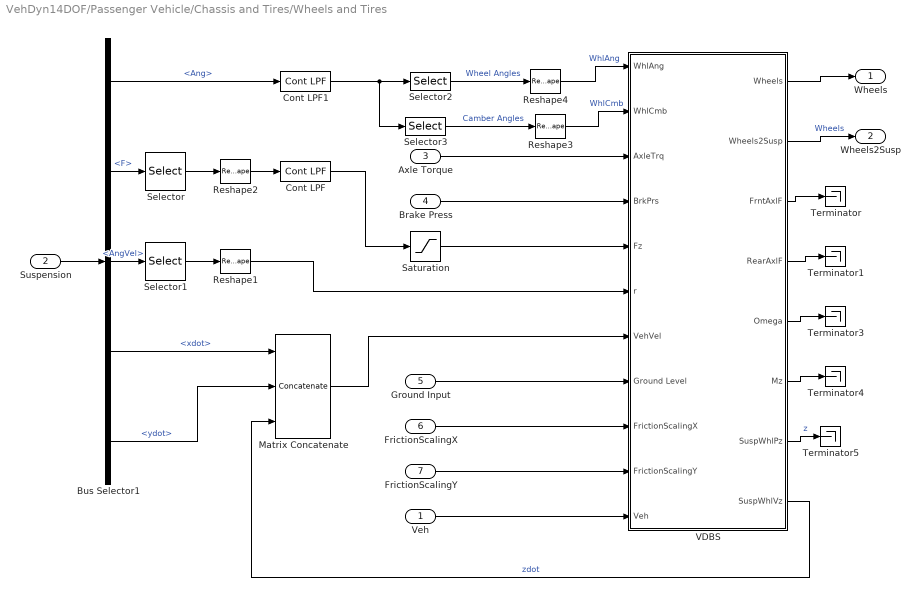
== system VehDyn14DOF/Passenger Vehicle/Chassis and Tires/Wheels and Tires ==
  Veh : Inport
  Suspension : Inport  Port=2
  Axle Torque : Inport  Port=3
  Brake Press : Inport  Port=4  Unit=Pa
  Ground Input : Inport  Port=5
  FrictionScalingX : Inport  Port=6  Unit=1  PortDimensions=4
  FrictionScalingY : Inport  Port=7  Unit=1  PortDimensions=4
  Bus Selector1 : BusSelector  OutputSignals=Whl.Ang,Whl.F,Whl.AngVel,Whl.xdot,Whl.ydot
  Cont LPF : autolibutils/Cont LPF  wc=100*2*pi  AbsoluteTolerance=auto  aMode=2
  Cont LPF1 : autolibutils/Cont LPF  wc=100*2*pi  AbsoluteTolerance=auto  aMode=2
  Matrix Concatenate : Concatenate  NumInputs=3  Mode=Multidimensional array
  Reshape{1..4} (4 alike) : Reshape
  Saturation : Saturate  UpperLimit=inf  LowerLimit=-10*9.81*2000  ZeroCross=off
  Selector : Selector  NumberOfDimensions=2  InputPortWidth=3  IndexOptions=Index vector (dialog),Select all  Indices=[3],1  OutputSizes=1,1
  Selector1 : Selector  NumberOfDimensions=2  InputPortWidth=1  IndexOptions=Index vector (dialog),Select all  Indices=[3],1  OutputSizes=1,1
  Selector2 : Selector  NumberOfDimensions=2  InputPortWidth=3  IndexOptions=Index vector (dialog),Select all  Indices=3,1  OutputSizes=1,1
  Selector3 : Selector  NumberOfDimensions=2  InputPortWidth=3  IndexOptions=Index vector (dialog),Select all  Indices=1,1  OutputSizes=1,1
  Terminator{,1,3..5} (5 alike) : Terminator
  VDBS : Subsystem  VariantControl=0
  Wheels : Outport  VectorParamsAs1DForOutWhenUnconnected=off
  Wheels2Susp : Outport  Port=2  VectorParamsAs1DForOutWhenUnconnected=off
  wires:
  Bus Selector1/2 -> Selector/1  "<F>"
  VDBS/3(FrntAxlF) -> Terminator/1
  VDBS/4(RearAxlF) -> Terminator1/1
  VDBS/5(Omega) -> Terminator3/1
  VDBS/6(Mz) -> Terminator4/1
  Selector1/1 -> Reshape1/1
  Matrix Concatenate/1 -> VDBS/7(VehVel)
  Axle Torque/1 -> VDBS/3(AxleTrq)
  Reshape4/1 -> VDBS/1(WhlAng)  "WhlAng"
  Reshape3/1 -> VDBS/2(WhlCmb)  "WhlCmb"
  Selector/1 -> Reshape2/1
  Saturation/1 -> VDBS/5(Fz)
  Ground Input/1 -> VDBS/8(Ground Level)
  VDBS/8(SuspWhlVz) -> Matrix Concatenate/3  "zdot"
  Bus Selector1/1 -> Cont LPF1/1  "<Ang>"
  Selector3/1 -> Reshape3/1  "Camber Angles"
  Suspension/1 -> Bus Selector1/1
  Bus Selector1/4 -> Matrix Concatenate/1  "<xdot>"
  Bus Selector1/5 -> Matrix Concatenate/2  "<ydot>"
  VDBS/7(SuspWhlPz) -> Terminator5/1  "z"
  Reshape2/1 -> Cont LPF/1
  Bus Selector1/3 -> Selector1/1  "<AngVel>"
  Reshape1/1 -> VDBS/6(r)
  Brake Press/1 -> VDBS/4(BrkPrs)
  FrictionScalingX/1 -> VDBS/9(FrictionScalingX)
  Cont LPF/1 -> Saturation/1
  Cont LPF1/1 -> Selector3/1, Selector2/1
  Selector2/1 -> Reshape4/1  "Wheel Angles"
  Veh/1 -> VDBS/11(Veh)
  VDBS/2(Wheels2Susp) -> Wheels2Susp/1  "Wheels"
  VDBS/1(Wheels) -> Wheels/1
  FrictionScalingY/1 -> VDBS/10(FrictionScalingY)

== system VehDyn14DOF/Passenger Vehicle/Engine/Accessory Load Model ==
  EngTrqIn : Inport
  EngSpd : Inport  Port=2
  Accessory Load Power : Lookup_n-D  NumberOfTableDimensions=1  LookupTableObject=''  BreakpointsForDimension1=AccSpdbp  Table=AccPwrbp  ExtrapMethod=Clip  InternalRulePriority=Speed  RndMeth=Simplest
  Divide : Product  Inputs=*/
  Kw to w : Gain  Gain=1000
  Net Torque : Sum  Inputs=+-
  Saturation : Saturate  UpperLimit=Inf  LowerLimit=300
  rpm to rad/s : Gain  Gain=pi/30
  EngTrqOut : Outport  Unit=N*m  VectorParamsAs1DForOutWhenUnconnected=off
  wires:
  Divide/1 -> Net Torque/2
  Accessory Load Power/1 -> Kw to w/1
  EngSpd/1 -> Saturation/1, Accessory Load Power/1
  Saturation/1 -> rpm to rad/s/1
  rpm to rad/s/1 -> Divide/2
  Net Torque/1 -> EngTrqOut/1
  Kw to w/1 -> Divide/1
  EngTrqIn/1 -> Net Torque/1

== system VehDyn14DOF/Passenger Vehicle/Pedal Cluster and Cabin/Brake Pedal ==
  DecelCmd : Inport
  Constant1 : Constant  Value=-20
  Dead Zone1 : DeadZone  LowerValue=0  UpperValue=.01  ZeroCross=off
  Gain3 : Gain
  Integrator2 : Integrator  LimitOutput=on  UpperSaturationLimit=1  LowerSaturationLimit=0
  Switch1 : Switch  Criteria=u2 > Threshold  Threshold=.1  SaturateOnIntegerOverflow=off  InputSameDT=off
  DecelFdbk : Outport
  wires:
  Dead Zone1/1 -> Switch1/2, Gain3/1
  Constant1/1 -> Switch1/3
  Integrator2/1 -> DecelFdbk/1
  Gain3/1 -> Switch1/1
  Switch1/1 -> Integrator2/1
  DecelCmd/1 -> Dead Zone1/1

== system VehDyn14DOF/Passenger Vehicle/Steering and Driveline/Brake Hydraulics ==
  BrkPrsCmd : Inport
  Dead Zone : DeadZone  LowerValue=-inf  UpperValue=1e-3  ZeroCross=off
  Front Bias : Constant
  Gain4 : Gain  Gain=8e6
  Mux : Mux
  Product : Product
  Rear Bias : Constant  Value=.6
  Valve : autolibutils/Cont LPF  wc=40*pi  AbsoluteTolerance=auto  aMode=2
  BrkPrs : Outport  VectorParamsAs1DForOutWhenUnconnected=off
  wires:
  Dead Zone/1 -> Valve/1
  Valve/1 -> Product/2  "Flow"
  Gain4/1 -> BrkPrs/1
  BrkPrsCmd/1 -> Dead Zone/1
  Front Bias/1 -> Mux/2, Mux/1
  Rear Bias/1 -> Mux/3, Mux/4
  Product/1 -> Gain4/1
  Mux/1 -> Product/1

== system VehDyn14DOF/Passenger Vehicle/Steering and Driveline/Driveline Model ==
  DrvShfTrq : Inport
  Omega : Inport  Port=2
  DiffPrsCmd : Inport  Port=3
  All Wheel Drive : Subsystem  VariantControl=2
  Front Wheel Drive : Subsystem  VariantControl=1
  Rear Wheel Drive : Subsystem  VariantControl=0
  Rear Wheel Drive Active Differential : Subsystem  VariantControl=4
  AxlTrq : Outport  VectorParamsAs1DForOutWhenUnconnected=off
  PropShaftSpd : Outport  Port=2  VectorParamsAs1DForOutWhenUnconnected=off

== system VehDyn14DOF/Passenger Vehicle/Steering and Driveline/Transmission ==
  GearCmd : Inport
  EngTrq : Inport  Port=2
  PropShftSpd : Inport  Port=3
  Ideal : Subsystem  VariantControl=0
  Info : Outport  VectorParamsAs1DForOutWhenUnconnected=off
  EngSpd : Outport  Port=2  VectorParamsAs1DForOutWhenUnconnected=off
  DrvShfTrq : Outport  Port=3  VectorParamsAs1DForOutWhenUnconnected=off

== system VehDyn14DOF/Controllers/Brake Pressure Control/Bang Bang ABS/Bang-bang controller ==
  in_1 : Inport
  Constant : Constant  Value=0
  Data Type Conversion1 : DataTypeConversion  OutDataTypeStr=double
  Data Type Conversion2 : DataTypeConversion  OutDataTypeStr=double
  Relational Operator : RelationalOperator  Operator=>  OutDataTypeStr=boolean
  Relational Operator1 : RelationalOperator  Operator=<  OutDataTypeStr=boolean
  Sum : Sum  Inputs=+-  InputSameDT=on  SaturateOnIntegerOverflow=on  OutDataTypeStr=Inherit: Same as first input
  out_1 : Outport  InitialOutput=0  VectorParamsAs1DForOutWhenUnconnected=off
  wires:
  Data Type Conversion2/1 -> Sum/2
  Data Type Conversion1/1 -> Sum/1
  Sum/1 -> out_1/1
  Relational Operator/1 -> Data Type Conversion1/1
  Relational Operator1/1 -> Data Type Conversion2/1
  Constant/1 -> Relational Operator/2, Relational Operator1/2
  in_1/1 -> Relational Operator1/1, Relational Operator/1

== system VehDyn14DOF/Controllers/Brake Pressure Control/Bang Bang ABS/Kappa ==
  xdot : Inport
  Omega : Inport  Port=2  Partition=on  PartitionDimension=1  PartitionWidth=1  PartitionOffset=0
  For Each : ForEach  DisableCoverage=on
  MATLAB Function : MATLAB Function  TreatAsAtomicUnit=on
  KappaEst : Outport  ConcatenationDimension=1
  wires:
  MATLAB Function/1(KappaEst) -> KappaEst/1
  xdot/1 -> MATLAB Function/2(xdot)
  Omega/1 -> MATLAB Function/1(Omega)

== system VehDyn14DOF/Controllers/Brake Pressure Control/Five-State ABS/ABSCtrlForEach ==
  Pref : Inport
  WhlAccel : Inport  Port=2
  WhlSlip : Inport  Port=3
  VehSpd : Inport  Port=4
  Constant7 : Constant  Value=WhlAccelOpt
  Constant8 : Constant  Value=KappaOpt
  For Each Subsystem : Subsystem  TreatAsAtomicUnit=on
  Gain : Gain  Gain=Re
  Saturation1 : Saturate  UpperLimit=1  LowerLimit=-1
  Selector : Selector  InputPortWidth=1  IndexOptions=Index vector (dialog)  Indices=[1 1 1 1]  OutputSizes=1
  Sum : Sum  Inputs=|+-
  Sum1 : Sum  Inputs=|+-
  BrkCtrl : Outport
  BrkFlag : Outport  Port=2
  wires:
  Gain/1 -> Sum/1
  Constant8/1 -> Sum1/2
  WhlSlip/1 -> Saturation1/1
  Constant7/1 -> Sum/2
  Sum1/1 -> For Each Subsystem/1(e1)
  WhlAccel/1 -> Gain/1
  Saturation1/1 -> Sum1/1
  For Each Subsystem/2(Flag) -> BrkFlag/1
  Pref/1 -> Selector/1
  VehSpd/1 -> For Each Subsystem/4(VehSpd)
  For Each Subsystem/1(Pb) -> BrkCtrl/1  "BrkPrsCmdCtrl"
  Selector/1 -> For Each Subsystem/3(Pref)
  Sum/1 -> For Each Subsystem/2(e2)

== system VehDyn14DOF/Controllers/Brake Pressure Control/Five-State ABS/Wheel Accel and Slip Estimator ==
  Omega : Inport
  Accel : Inport  Port=2
  Demux : Demux  Outputs=3
  Discrete-Time Integrator : DiscreteIntegrator  IntegratorMethod=Integration: Trapezoidal  SampleTime=-1  ICPrevOutput=DiscIntNeverNeededParam  ICPrevScaledInput=DiscIntNeverNeededParam
  Kappa : Subsystem  TreatAsAtomicUnit=on
  Terminator : Terminator
  Terminator1 : Terminator
  Wheel Accel : Subsystem  TreatAsAtomicUnit=on
  <WhlAccel> : Outport
  <Kappa> : Outport  Port=2
  <xdot> : Outport  Port=3
  wires:
  Accel/1 -> Demux/1
  Discrete-Time Integrator/1 -> <xdot>/1, Kappa/1(xdot)
  Demux/1 -> Discrete-Time Integrator/1
  Demux/2 -> Terminator/1
  Demux/3 -> Terminator1/1
  Omega/1 -> Kappa/2(Omega), Wheel Accel/1(Omega)
  Wheel Accel/1(WhlAccel) -> <WhlAccel>/1
  Kappa/1(KappaEst) -> <Kappa>/1

== system VehDyn14DOF/Controllers/ECU/Torque Cmd/Rev Limiter Control ==
  TrqCmd : Inport
  EngSpd : Inport  Port=2
  1-D Lookup Table : Lookup_n-D  NumberOfTableDimensions=1  BreakpointsForDimension1=[1 1.01]  Table=[1 0]  ExtrapMethod=Clip  InternalRulePriority=Speed  RndMeth=Simplest
  Constant : Constant  Value=EngRevLim
  Product : Product
  Product1 : Product  Inputs=*/
  TrqCmdRevLimited : Outport  VectorParamsAs1DForOutWhenUnconnected=off
  wires:
  EngSpd/1 -> Product1/1
  Product/1 -> TrqCmdRevLimited/1
  1-D Lookup Table/1 -> Product/2
  TrqCmd/1 -> Product/1
  Constant/1 -> Product1/2
  Product1/1 -> 1-D Lookup Table/1

== system VehDyn14DOF/Controllers/Transmission Controller/Transmission Controller/TCM ==
  AccCmd : Inport
  EngSpd : Inport  Port=2
  Omega : Inport  Port=3  Unit=rad/s
  function : TriggerPort  TriggerType=function-call  VariantControl=Variant
  Gain : Gain  Gain=.3065/4
  Neutral Select : Subsystem
  Signal Specification1 : SignalSpecification  Unit=m/s
  Signal Specification2 : SignalSpecification  Unit=km/hr
  Speed LPF : DiscreteTransferFcn  Numerator=[0.000000000000000 0.009950166250832 ]  Denominator=[1.000000000000000 -0.990049833749168 ]  mask(DiscretizedDiscreteTransferFcn){}
      mask init:
      | %zoh
  Sum of Elements : Sum  Inputs=+
  TCM Shift Controller : Stateflow chart  TreatAsAtomicUnit=on
  Unit Conversion1 : UnitConversion
  GearCmd : Outport  VectorParamsAs1DForOutWhenUnconnected=off
  wires:
  Signal Specification2/1 -> Speed LPF/1
  TCM Shift Controller/1(GearCmd) -> GearCmd/1  "GearCmd"
  AccCmd/1 -> Neutral Select/1(AccCmd), TCM Shift Controller/2(pedal)  "AccCmd"
  Neutral Select/1(Neutral Select) -> TCM Shift Controller/3(Neutral)
  EngSpd/1 -> Neutral Select/2(EngSpd)
  Speed LPF/1 -> TCM Shift Controller/1(speed)
  Unit Conversion1/1 -> Signal Specification2/1
  Omega/1 -> Sum of Elements/1
  Gain/1 -> Signal Specification1/1
  Signal Specification1/1 -> Unit Conversion1/1
  Sum of Elements/1 -> Gain/1

== system VehDyn14DOF/Passenger Vehicle/Chassis and Tires/Suspension/Double Wishbone Suspension ==
  Wheel : Inport
  Steering : Inport  Port=2
  Vehicle : Inport  Port=3
  Bus Creator1 : BusCreator  Inputs=6
  Bus Creator2 : BusCreator  Inputs=2
  Bus Creator3 : BusCreator  Inputs=2
  Bus Creator4 : BusCreator  Inputs=6
  Bus Selector : BusSelector  OutputSignals=z,Re,zdot,Fx,Fy,M
  Bus Selector1 : BusSelector  OutputSignals=P,V
  Bus Selector2 : BusSelector  OutputSignals=SuspFrame.z
  Independent Suspension – Double Wishbone : vehdynlibsuspension/Independent Suspension - Double Wishbone  ActiveDampEn=off  NumAxl=2  NumWhlsByAxl=[2 2]  StrgEnByAxl=[1 0]  AntiSwayEnByAxl=[1 0]  WhlNumVec="[1  2  1  2]"  AxleNumVec="[1  1  2  2]"  SuspTypesByAxle="[1  1]"  SuspImage=suspdw.png  IdealSuspEn=on  IdealSuspAxles="[1  2]"  Kz=Kz  F0z=F0z  Cz=Cz  Hmax=Hmax  f_act_susp_cz=[10000 10000;10000 10000]  f_act_susp_duty_bpt=[0 1]  f_act_susp_zdot_bpt=[-1 1]  Toe=0.  RollStrgSlp=0.  ToeStrgSlp=0.  Caster=0.  CasterHslp=0.  CasterStrgSlp=0.  Camber=0.  CamberHslp=0.  CamberStrgSlp=0.  StrgHgtSlp=0.1432  MappedSuspEn=off  MappedSuspAxles="[1  2]"  f_susp_axl_bp=[1 2]  f_susp_dz_bp=[-0.15 -0.14 -0.13 -0.12 -0.11 -0.10 -0.09 -0.08 -0.07 -0.06 -0.05 -0.04 -0.03 -0.02 -0.01 0.00 0.01 0.02 0.03 0.04 0.05 0.06 0.07 0.08 0.09 0.10 0.11 0.12 0.13 0.14 0.15]  f_susp_dzdot_bp=[-0.15 -0.14 -0.13 -0.12 -0.11 -0.10 -0.09 -0.08 -0.07 -0.06 -0.05 -0.04 -0.03 -0.02 -0.01 0.00 0.01 0.02 0.03 0.04 0.05 0.06 0.07 0.08 0.09 0.10 0.11 0.12 0.13 0.14 0.15]  f_susp_fmz=zeros(31,31,61,2,4)  f_susp_geom=zeros(31,61,2,3)  f_susp_strgdelta_bp=[-30,-29,-28,-27,-26,-25,-24,-23,-22,-21,-20,-19,-18,-17,-16,-15,-14,-13,-12,-11,-10,-9,-8,-7,-6,-5,-4,-3,-2,-1,0,1,2,3,4,5,6,7,8,9,10,11,12,13,14,15,16,17,18,19,20,21,22,23,24,25,26,27,28,29,30]  AntiSwayR=0.2  AntiSwayNtrlAng=0.5236  AntiSwayTrsK=8e2
  Selector1 : Selector  NumberOfDimensions=2  IndexOptions=Index vector (dialog),Select all  Indices=1,1  OutputSizes=1,1
  Selector2 : Selector  NumberOfDimensions=2  IndexOptions=Index vector (dialog),Select all  Indices=2,1  OutputSizes=1,1
  Steer Rate Adapter : Subsystem
  Steering Adapter : Subsystem
  Terminator : Terminator
  Terminator1 : Terminator
  Vehicle Adapter : Subsystem
  Wheel  Adapter : Subsystem
  Wheel1 : InportShadow
  Suspension : Outport  VectorParamsAs1DForOutWhenUnconnected=off
  wires:
  Bus Creator3/1 -> Suspension/1
  Steering Adapter/1(StrgAng) -> Independent Suspension – Double Wishbone/9
  Independent Suspension – Double Wishbone/1 -> Terminator/1
  Wheel  Adapter/6(Re) -> Bus Creator4/6
  Bus Selector1/1 -> Independent Suspension – Double Wishbone/7  "<P>"
  Wheel  Adapter/2(WhlFy) -> Bus Creator4/2  "Fy"
  Wheel/1 -> Wheel  Adapter/1(Wheels)
  Steer Rate Adapter/1(AngVel) -> Bus Creator1/6  "AngVel"
  Bus Creator4/1 -> Bus Selector/1
  Bus Creator2/1 -> Bus Creator3/1  "Veh"
  Vehicle Adapter/2(VehVbody) -> Selector1/1, Selector2/1  "V"
  Selector2/1 -> Bus Creator1/3  "ydot"
  Bus Selector1/2 -> Independent Suspension – Double Wishbone/8  "<V>"
  Independent Suspension – Double Wishbone/2 -> Bus Creator2/1  "F"
  Bus Selector/2 -> Independent Suspension – Double Wishbone/2  "<Re>"
  Wheel  Adapter/5(M) -> Bus Creator4/5  "M"
  Bus Selector/4 -> Independent Suspension – Double Wishbone/4  "<Fx>"
  Independent Suspension – Double Wishbone/4 -> Bus Creator1/1  "F"
  Steering/1 -> Steering Adapter/1(Steer)
  Selector1/1 -> Bus Creator1/2  "xdot"
  Independent Suspension – Double Wishbone/3 -> Bus Creator2/2  "M"
  Vehicle Adapter/1(VehSusp) -> Bus Selector1/1
  Wheel  Adapter/4(zdot) -> Bus Creator4/4
  Vehicle/1 -> Vehicle Adapter/1(Veh), Steer Rate Adapter/1(Veh)
  Bus Selector/6 -> Independent Suspension – Double Wishbone/6  "<M>"
  Bus Selector/5 -> Independent Suspension – Double Wishbone/5  "<Fy>"
  Bus Selector/1 -> Independent Suspension – Double Wishbone/1  "<z>"
  Wheel  Adapter/3(z) -> Bus Creator4/3
  Independent Suspension – Double Wishbone/6 -> Bus Creator1/4  "Ang"
  Bus Creator1/1 -> Bus Creator3/2  "Whl"
  Wheel  Adapter/1(WhlFx) -> Bus Creator4/1  "Fx"
  Bus Selector/3 -> Independent Suspension – Double Wishbone/3  "<zdot>"
  Independent Suspension – Double Wishbone/5 -> Terminator1/1  "V"
  Bus Selector2/1 -> Bus Creator1/5  "<z>"
  Wheel1/1 -> Bus Selector2/1
